simulink model "fourmasses"  (Simulink 7.9)
settings: Solver=ode45  StartTime=0.0  StopTime=60  RelTol=1e-3
values from neighbouring files (symbols this model uses):
  A = params.A    [cvxsolve.m]
  B = params.B    [cvxsolve.m]
  bd = [kron(ones(T,1),eye(n))]    [prepFourMasses.m]    (also in prepSixMasses.m; prepSoftKS.m)
  bx = [A; zeros(ellef+(T-1)*n,n)]    [prepFourMasses.m]    (also in prepSixMasses.m; prepSoftKS.m)
  C = [kron(eye(T),[-B eye(n)]) + kron([zeros(1,T); eye(T-1) zeros(T-1,1)],[zeros(n,m) -A]); zeros(ellef,m+(T-1)*(m+n)) Ef]    [prepFourMasses.m]    (also in prepSixMasses.m; prepSoftKS.m)
  dt = 0.5    [prepFourMasses.m]    (also in prepSixMasses.m; prepSoftKS.m)
  Ef_block = zeros(2*n,1)    [prepFourMasses.m]    (also in prepSixMasses.m; prepSoftKS.m)
  Ff = params.Ff    [cvxsolve.m]    (also in prepFourMasses.m = [[1] zeros(1,7)]; prepSixMasses.m = [[1;1] zeros(2,11)]; prepSoftKS.m = [[1;1] zeros(2,11)])
  Fu = params.Fu    [cvxsolve.m]    (also in prepFourMasses.m = [eye(2); -eye(2) ]; prepSixMasses.m = [eye(3); -eye(3) ]; prepSoftKS.m = [eye(3); -eye(3) ])
  Fus = [zeros(4,2)]    [prepFourMasses.m]    (also in prepSixMasses.m = [zeros(12,3)]; prepSoftKS.m = [zeros(12,3)])
  Fx = [zeros(4,8)]    [prepFourMasses.m]    (also in prepSixMasses.m = [zeros(6,12)]; prepSoftKS.m = [zeros(6,12)])
  Fxs = params.Fxs    [cvxsolve.m]    (also in prepFourMasses.m = [eye(4) zeros(4)]*100; prepSixMasses.m = [eye(6) zeros(6); prepSoftKS.m = [eye(6) zeros(6))
  g = [r; repmat([q;r],T-1,1); qf]    [prepFourMasses.m]    (also in prepSixMasses.m; prepSoftKS.m)
  H = blkdiag(R,kron(eye(T-1),blkdiag(Q,R)),Qf)    [prepFourMasses.m]    (also in prepSixMasses.m; prepSoftKS.m)
  hc = [repmat(f,T,1);ff]    [prepFourMasses.m]    (also in prepSixMasses.m; prepSoftKS.m)
  hcs = [repmat(fs,T,1)]    [prepFourMasses.m]    (also in prepSixMasses.m; prepSoftKS.m)
  hx = [-Fx; zeros((T-1)*ell + ellf,n)]    [prepFourMasses.m]    (also in prepSixMasses.m; prepSoftKS.m)
  hxs = [-Fxs; zeros((T-1)*ells,n)]    [prepFourMasses.m]    (also in prepSixMasses.m; prepSoftKS.m)
  m = size(B,2)    [prepFourMasses.m]    (also in prepSixMasses.m; prepSoftKS.m)
  n = size(A,1)    [prepFourMasses.m]    (also in prepSixMasses.m; prepSoftKS.m)
  opts = []    [prepFourMasses.m]    (also in prepSixMasses.m; prepSoftKS.m)
  P = blkdiag(Fu,kron(eye(T-1),[Fx Fu]),Ff)    [prepFourMasses.m]    (also in prepSixMasses.m; prepSoftKS.m)
  Ps = blkdiag(Fus,kron(eye(T-1),[Fxs Fus]))    [prepFourMasses.m]    (also in prepSixMasses.m; prepSoftKS.m)
  Q = params.Q    [cvxsolve.m]    (also in prepFourMasses.m = eye(8); prepSixMasses.m = eye(12); prepSoftKS.m = eye(12))
  R = params.R    [cvxsolve.m]    (also in prepFourMasses.m = eye(2); prepSixMasses.m = eye(3); prepSoftKS.m = eye(3))
  T = 11    [prepFourMasses.m]    (also in prepSixMasses.m = 31; prepSoftKS.m = 10)
undefined symbols (not defined in the file or in its folder): Qf
settings Model: Creator=aeagr  LastModifiedBy=aeagr

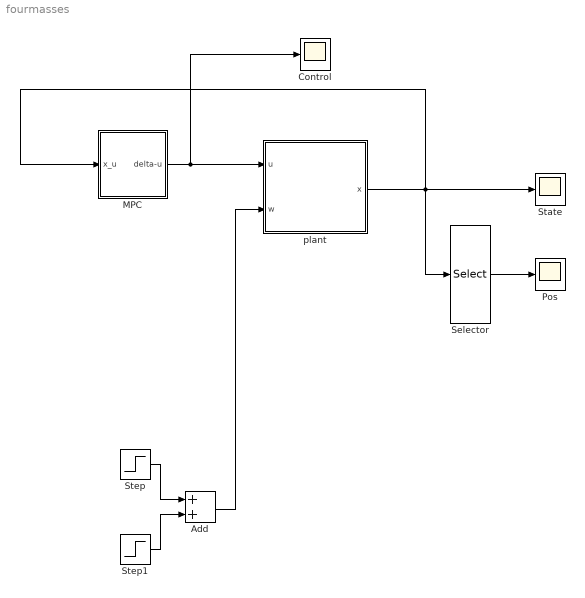
== system fourmasses ==
  Add : Sum
  Control : Scope
      settings: TimeRange=60  YMin=-0.5  YMax=0.5
  MPC : Subsystem  RequirementInfo={} %GIDa_c7b45cd4_27da_4c63_877d_a3adaac8971e  TreatAsAtomicUnit=on  SystemSampleTime=dt
      settings: RTWSystemCode=Function  RTWFcnNameOpts=Use subsystem name  RTWFileNameOpts=Use subsystem name
  Pos : Scope
      settings: YMin=-0.7  YMax=0.8  SaveName=ScopeData2
  Selector : Selector  InputPortWidth=8  IndexOptions=Index vector (dialog)  Indices=[1:4]  OutputSizes=1
  State : Scope
      settings: YMin=-0.7  YMax=0.8
  Step : Step  Time=10  Before=zeros(4,1)  After=[0.5;0;0;0]  SampleTime=0
  Step1 : Step  Time=30  Before=zeros(4,1)  After=-[0.5;0;0;0]  SampleTime=0
  plant : Subsystem
  wires:
  MPC/1(delta-u) -> plant/1(u), Control/1
  plant/1(x) -> State/1, Selector/1, MPC/1(x_u)
  Selector/1 -> Pos/1
  Step1/1 -> Add/2
  Step/1 -> Add/1
  Add/1 -> plant/2(w)

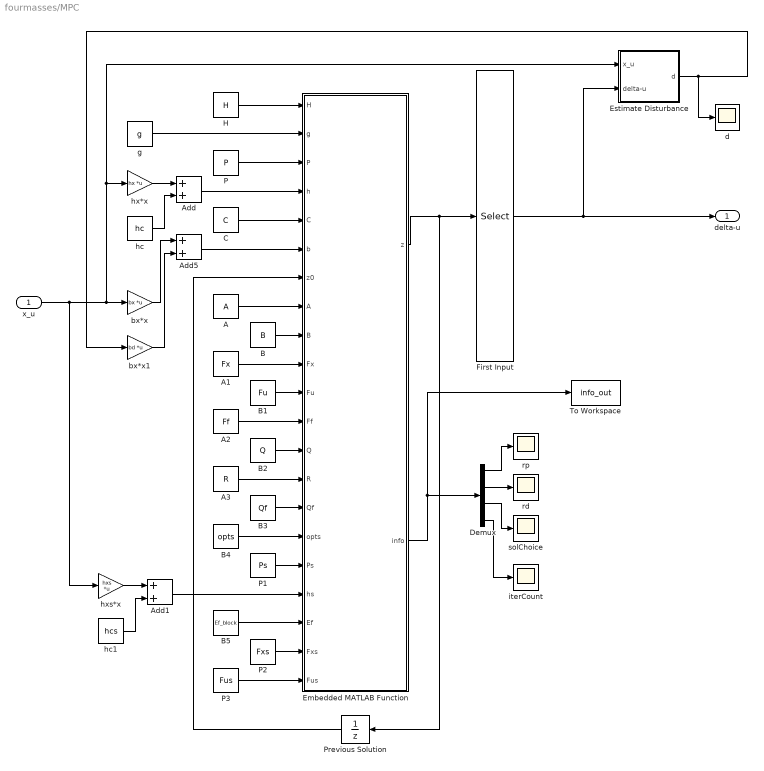
== system fourmasses/MPC ==
  x_u : Inport
  A : Constant  Value=A
  A1 : Constant  Value=Fx
  A2 : Constant  Value=Ff  VectorParams1D=off
  A3 : Constant  Value=R
  Add : Sum
  Add1 : Sum
  Add5 : Sum
  B : Constant  Value=B
  B1 : Constant  Value=Fu
  B2 : Constant  Value=Q
  B3 : Constant  Value=Qf
  B4 : Constant  Value=opts
  B5 : Constant  Value=Ef_block
  C : Constant  Value=C
  Demux : Demux
  Embedded MATLAB Function : MATLAB Function  TreatAsAtomicUnit=on
      settings: RTWFileNameOpts=Use subsystem name
  Estimate Disturbance : Subsystem
  First Input : Selector  InputPortWidth=T*(n+m)  IndexOptions=Index vector (dialog)  Indices=1:2  OutputSizes=1
  H : Constant  Value=H
  P : Constant  Value=P
  P1 : Constant  Value=Ps
  P2 : Constant  Value=Fxs
  P3 : Constant  Value=Fus
  Previous Solution : UnitDelay  SampleTime=-1
  To Workspace : ToWorkspace  VariableName=info_out  SampleTime=-1
  bx*x : Gain  Gain=bx  Multiplication=Matrix(K*u)
  bx*x1 : Gain  Gain=bd  Multiplication=Matrix(K*u)
  d : Scope
      settings: YMin=-0.025  YMax=0.25  SaveName=ScopeData6
  g : Constant  Value=g
  hc : Constant  Value=hc
  hc1 : Constant  Value=hcs
  hx*x : Gain  Gain=hx  Multiplication=Matrix(K*u)
  hxs*x : Gain  Gain=hxs  Multiplication=Matrix(K*u)
  iterCount : Scope
      settings: TimeRange=60  YMin=0  YMax=100  SaveName=ScopeData9
  rd : Scope
      settings: YMin=0  YMax=375  SaveName=ScopeData4
  rp : Scope
      settings: YMin=-0.05  YMax=0.65  SaveName=ScopeData3
  solChoice : Scope
      settings: YMin=0.95  YMax=1.05  SaveName=ScopeData5
  delta-u : Outport
  wires:
  First Input/1 -> delta-u/1, Estimate Disturbance/2(delta-u)
  Embedded MATLAB Function/1(z) -> Previous Solution/1, First Input/1
  Previous Solution/1 -> Embedded MATLAB Function/7(z0)
  H/1 -> Embedded MATLAB Function/1(H)
  P/1 -> Embedded MATLAB Function/3(P)
  C/1 -> Embedded MATLAB Function/5(C)
  Add/1 -> Embedded MATLAB Function/4(h)
  x_u/1 -> bx*x/1, hx*x/1, Estimate Disturbance/1(x_u), hxs*x/1
  hx*x/1 -> Add/1
  hc/1 -> Add/2
  B/1 -> Embedded MATLAB Function/9(B)
  A/1 -> Embedded MATLAB Function/8(A)
  B3/1 -> Embedded MATLAB Function/15(Qf)
  A3/1 -> Embedded MATLAB Function/14(R)
  B2/1 -> Embedded MATLAB Function/13(Q)
  A2/1 -> Embedded MATLAB Function/12(Ff)
  B1/1 -> Embedded MATLAB Function/11(Fu)
  A1/1 -> Embedded MATLAB Function/10(Fx)
  Embedded MATLAB Function/2(info) -> Demux/1, To Workspace/1
  Demux/1 -> rp/1
  Demux/2 -> rd/1
  Demux/3 -> solChoice/1
  B4/1 -> Embedded MATLAB Function/16(opts)
  P1/1 -> Embedded MATLAB Function/17(Ps)
  hxs*x/1 -> Add1/1
  hc1/1 -> Add1/2
  Add1/1 -> Embedded MATLAB Function/18(hs)
  Estimate Disturbance/1(d) -> d/1, bx*x1/1
  g/1 -> Embedded MATLAB Function/2(g)
  Add5/1 -> Embedded MATLAB Function/6(b)
  bx*x/1 -> Add5/1
  bx*x1/1 -> Add5/2
  B5/1 -> Embedded MATLAB Function/19(Ef)
  P2/1 -> Embedded MATLAB Function/20(Fxs)
  P3/1 -> Embedded MATLAB Function/21(Fus)
  Demux/4 -> iterCount/1

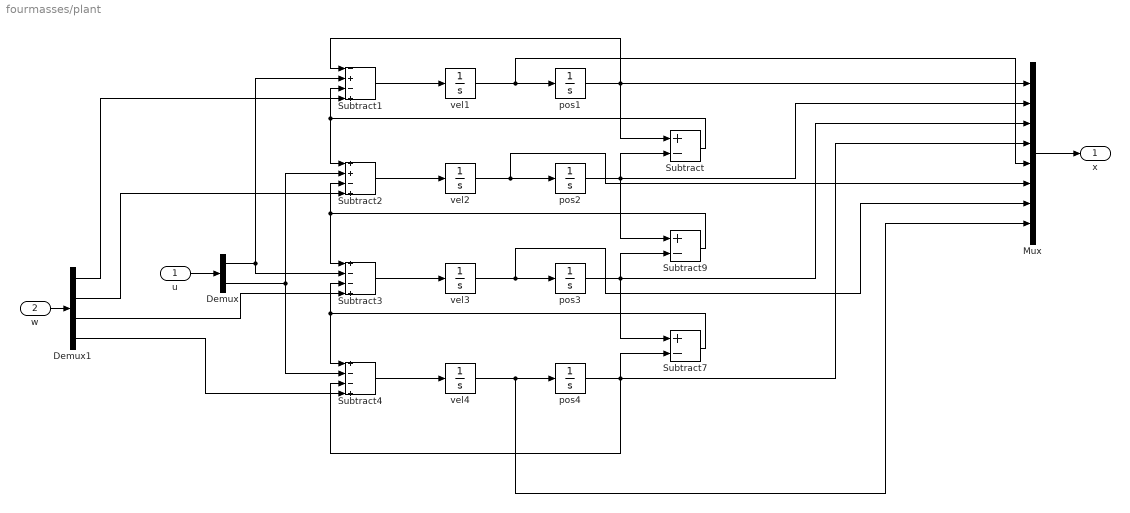
== system fourmasses/plant ==
  u : Inport
  w : Inport  Port=2
  Demux : Demux  Outputs=2
  Demux1 : Demux
  Mux : Mux  Inputs=8
  Subtract : Sum  Inputs=+-
  Subtract1 : Sum  Inputs=-+-+
  Subtract2 : Sum  Inputs=++-+
  Subtract3 : Sum  Inputs=+--+
  Subtract4 : Sum  Inputs=+--+
  Subtract7 : Sum  Inputs=+-
  Subtract9 : Sum  Inputs=+-
  pos{1..4} (4 alike) : Integrator
  vel{1..4} (4 alike) : Integrator
  x : Outport
  wires:
  vel1/1 -> pos1/1, Mux/5
  vel2/1 -> pos2/1, Mux/6
  vel3/1 -> pos3/1, Mux/7
  vel4/1 -> pos4/1, Mux/8
  pos1/1 -> Subtract/1, Subtract1/1, Mux/1
  pos2/1 -> Subtract/2, Subtract9/1, Mux/2
  pos3/1 -> Subtract7/1, Subtract9/2, Mux/3
  pos4/1 -> Subtract7/2, Mux/4, Subtract4/3
  Subtract/1 -> Subtract2/1, Subtract1/3
  Subtract9/1 -> Subtract3/1, Subtract2/3
  Subtract7/1 -> Subtract4/1, Subtract3/3
  Subtract4/1 -> vel4/1
  Subtract3/1 -> vel3/1
  Subtract2/1 -> vel2/1
  Subtract1/1 -> vel1/1
  Demux/1 -> Subtract1/2, Subtract3/2
  u/1 -> Demux/1
  Mux/1 -> x/1
  Demux1/3 -> Subtract3/4
  Demux1/4 -> Subtract4/4
  w/1 -> Demux1/1
  Demux1/1 -> Subtract1/4
  Demux1/2 -> Subtract2/4
  Demux/2 -> Subtract2/2, Subtract4/2

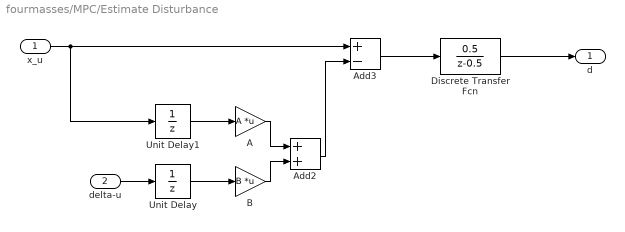
== system fourmasses/MPC/Estimate Disturbance ==
  x_u : Inport
  delta-u : Inport  Port=2
  A : Gain  Gain=A  Multiplication=Matrix(K*u)
  Add2 : Sum
  Add3 : Sum  Inputs=+-
  B : Gain  Gain=B  Multiplication=Matrix(K*u)
  Discrete Transfer Fcn : DiscreteTransferFcn  Numerator=[0.5]  Denominator=[1 -0.5]
  Unit Delay : UnitDelay  SampleTime=-1
  Unit Delay1 : UnitDelay  SampleTime=-1
  d : Outport
  wires:
  Unit Delay1/1 -> A/1
  Unit Delay/1 -> B/1
  A/1 -> Add2/1
  B/1 -> Add2/2
  Add2/1 -> Add3/2
  x_u/1 -> Unit Delay1/1, Add3/1
  delta-u/1 -> Unit Delay/1
  Add3/1 -> Discrete Transfer Fcn/1
  Discrete Transfer Fcn/1 -> d/1

== matlab function MPC/Embedded MATLAB Function ==
  data: H input double; z output double; g input double; P input double; h input double; C input double; b input double size=T*n+ellef; z0 input double; A input double; B input double; Fx input double; Fu input double; Ff input double; Q input double; R input double; Qf input double; info output double; opts input double; Ps input double; hs input double; Ef input double; Fxs input double; Fus input double
function [z,info] = mpcsolve_simk(H,g,P,h,C,b,z0,A,B,Fx,Fu,Ff,Q,R,Qf,opts,Ps,hs,Ef,Fxs,Fus)
%#codegen

% just call to the Matlab version
[z,info] = mpcsolve(H,g,P,h,C,b,z0,A,B,Fx,Fu,Ff,Q,R,Qf,opts,Ps,hs,Ef,Fxs,Fus);
